simulink model "RANNSMC"  (R2017a)
settings: Solver=VariableStepAuto  StartTime=0.0  StopTime=10.0  RelTol=1e-3
undefined symbols (not defined in the file or in its folder): a21, a22
libraries: simulink x1
settings Model: Creator=ASUS  LastModifiedBy=ASUS

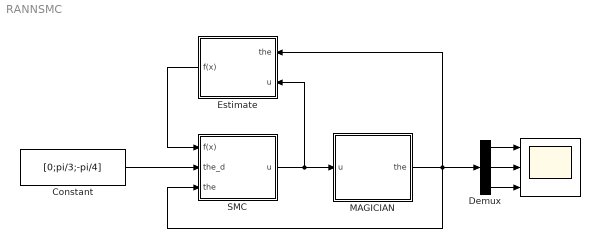
== system RANNSMC ==
  " " : Scope  NumInputPorts=3
  Constant : Constant  Value=[0;pi/3;-pi/4]
  Demux : Demux  Outputs=3
  Estimate : Subsystem
  MAGICIAN : Subsystem
  "SMC " : Subsystem
  wires:
  "SMC "/1("u ") -> MAGICIAN/1("u "), Estimate/2("u ")
  MAGICIAN/1(the) -> "SMC "/3("the "), Demux/1, Estimate/1(the)
  Demux/1 -> " "/1
  Demux/2 -> " "/2
  Demux/3 -> " "/3
  Estimate/1(f(x)) -> "SMC "/1(f(x))
  Constant/1 -> "SMC "/2(the_d)

== system RANNSMC/Estimate ==
  the : Inport
  "u " : Inport  Port=2
  Demux : Demux  Outputs=3
  Demux1 : Demux  Outputs=3
  Mux : Mux  Inputs=3
  "xx1 " : Subsystem
  "xx2 " : Subsystem
  xx3 : Subsystem
  f(x) : Outport
  wires:
  "u "/1 -> Demux1/1
  the/1 -> Demux/1
  Demux/1 -> "xx1 "/1(the1)
  Demux/2 -> "xx2 "/1(the2)
  Demux/3 -> xx3/1(the3)
  Demux1/1 -> "xx1 "/2(u1)
  Demux1/2 -> "xx2 "/2(u2)
  Demux1/3 -> xx3/2(u3)
  "xx1 "/1(f(x)1^) -> Mux/1
  xx3/1(f(x)3^) -> Mux/3
  Mux/1 -> f(x)/1
  "xx2 "/1(f(x)2^) -> Mux/2

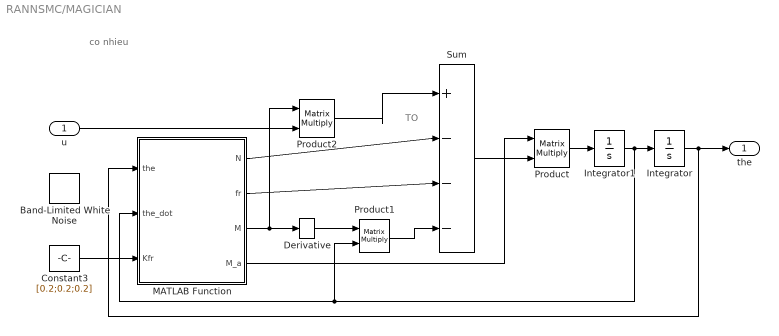
== system RANNSMC/MAGICIAN ==
  note: co nhieu
  note: TO
  "u " : Inport
  Band-Limited White Noise : simulink/Sources/Band-Limited White Noise  Cov=[0.1]  Ts=0.1  seed=[23341]
  Constant3 : Constant  Value=[0.2;0.2;0.2]
  Derivative : Derivative
  Integrator : Integrator  InitialCondition=[0;0;0]
  Integrator1 : Integrator  InitialCondition=[0;0;0]
  MATLAB Function : MATLAB Function  TreatAsAtomicUnit=on
  Product : Product  Multiplication=Matrix(*)
  Product1 : Product  Multiplication=Matrix(*)
  Product2 : Product  Multiplication=Matrix(*)
  Sum : Sum  Inputs=|+---
  the : Outport
  wires:
  Derivative/1 -> Product1/1
  Integrator1/1 -> MATLAB Function/2(the_dot), Product1/2, Integrator/1
  Product1/1 -> Sum/4
  Constant3/1 -> MATLAB Function/3(Kfr)
  MATLAB Function/3(M) -> Product2/1, Derivative/1
  Product/1 -> Integrator1/1
  MATLAB Function/2(fr) -> Sum/3
  MATLAB Function/1(N) -> Sum/2
  MATLAB Function/4(M_a) -> Product/1
  Integrator/1 -> MATLAB Function/1(the), the/1
  Sum/1 -> Product/2
  "u "/1 -> Product2/2
  Product2/1 -> Sum/1

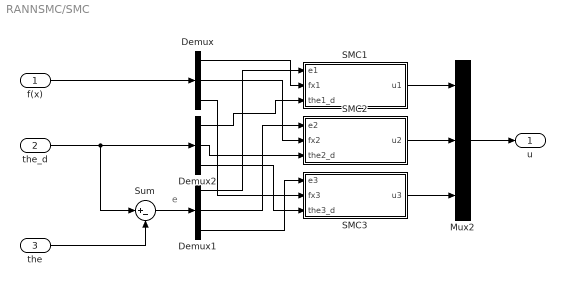
== system RANNSMC/SMC  ==
  note: e
  f(x) : Inport
  the_d : Inport  Port=2
  "the " : Inport  Port=3
  Demux : Demux  Outputs=3
  Demux1 : Demux  Outputs=3
  Demux2 : Demux  Outputs=3
  Mux2 : Mux  Inputs=3
  "SMC1 " : Subsystem
  "SMC2 " : Subsystem
  "SMC3 " : Subsystem
  Sum : Sum  Inputs=|+-
  "u " : Outport
  wires:
  "SMC1 "/1(u1) -> Mux2/1
  Mux2/1 -> "u "/1
  f(x)/1 -> Demux/1
  Demux/1 -> "SMC1 "/2(fx1)
  Demux1/1 -> "SMC1 "/1(e1)
  "SMC2 "/1(u2) -> Mux2/2
  Demux/2 -> "SMC2 "/2(fx2)
  Demux1/2 -> "SMC2 "/1(e2)
  the_d/1 -> Sum/1, Demux2/1
  Demux2/1 -> "SMC1 "/3(the1_d)
  "SMC3 "/1(u3) -> Mux2/3
  Demux1/3 -> "SMC3 "/1(e3)
  Demux/3 -> "SMC3 "/2(fx3)
  Demux2/2 -> "SMC2 "/3(the2_d)
  Demux2/3 -> "SMC3 "/3(the3_d)
  Sum/1 -> Demux1/1
  "the "/1 -> Sum/2

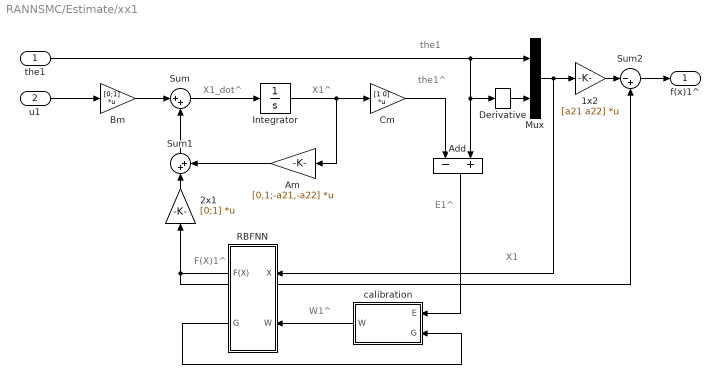
== system RANNSMC/Estimate/xx1  ==
  note: W1^
  note: the1
  note: the1^
  note: E1^
  note: X1_dot^
  note: X1^
  note: X1
  note: F(X)1^
  the1 : Inport
  u1 : Inport  Port=2
  " calibration" : Subsystem
  " RBFNN" : Subsystem
  1x2 : Gain  Gain=[a21 a22]  Multiplication=Matrix(K*u)
  2x1 : Gain  Gain=[0;1]  Multiplication=Matrix(K*u)
  Add : Sum  Inputs=-+
  "Am " : Gain  Gain=[0,1;-a21,-a22]  Multiplication=Matrix(K*u)
  Bm : Gain  Gain=[0;1]  Multiplication=Matrix(K*u)
  Cm : Gain  Gain=[1 0]  Multiplication=Matrix(K*u)
  Derivative : Derivative
  Integrator : Integrator
  Mux : Mux  Inputs=2
  Sum : Sum  Inputs=|++
  Sum1 : Sum  Inputs=|++
  Sum2 : Sum  Inputs=|-+
  f(x)1^ : Outport
  wires:
  Mux/1 -> 1x2/1, " RBFNN"/1("X ")
  Sum1/1 -> Sum/2
  u1/1 -> Bm/1
  2x1/1 -> Sum1/1
  Derivative/1 -> Mux/2
  Add/1 -> " calibration"/1(E)
  Sum/1 -> Integrator/1
  the1/1 -> Mux/1, Derivative/1, Add/2
  " calibration"/1(W) -> " RBFNN"/2(W)
  Integrator/1 -> Cm/1, "Am "/1
  "Am "/1 -> Sum1/2
  Sum2/1 -> f(x)1^/1
  " RBFNN"/2(G) -> " calibration"/2(G)
  Cm/1 -> Add/1
  1x2/1 -> Sum2/1
  Bm/1 -> Sum/1
  " RBFNN"/1(F(X)) -> 2x1/1, Sum2/2

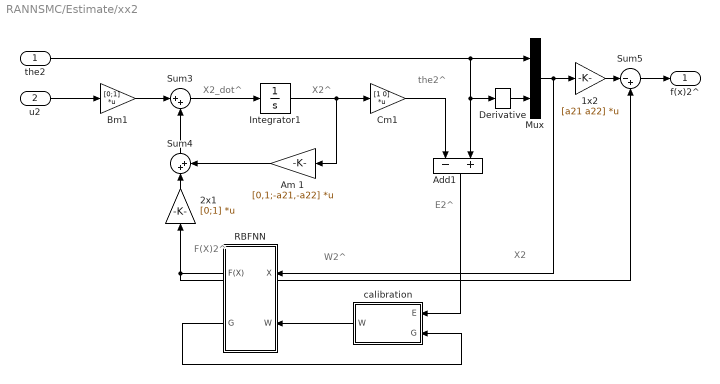
== system RANNSMC/Estimate/xx2  ==
  note: W2^
  note: the2^
  note: E2^
  note: X2_dot^
  note: X2^
  note: X2
  note: F(X)2^
  the2 : Inport
  u2 : Inport  Port=2
  " calibration" : Subsystem
  " RBFNN" : Subsystem
  1x2 : Gain  Gain=[a21 a22]  Multiplication=Matrix(K*u)
  2x1 : Gain  Gain=[0;1]  Multiplication=Matrix(K*u)
  Add1 : Sum  Inputs=-+
  Am 1 : Gain  Gain=[0,1;-a21,-a22]  Multiplication=Matrix(K*u)
  Bm1 : Gain  Gain=[0;1]  Multiplication=Matrix(K*u)
  Cm1 : Gain  Gain=[1 0]  Multiplication=Matrix(K*u)
  Derivative : Derivative
  Integrator1 : Integrator
  Mux : Mux  Inputs=2
  Sum3 : Sum  Inputs=|++
  Sum4 : Sum  Inputs=|++
  Sum5 : Sum  Inputs=|-+
  f(x)2^ : Outport
  wires:
  Mux/1 -> 1x2/1, " RBFNN"/1("X ")
  Sum4/1 -> Sum3/2
  u2/1 -> Bm1/1
  2x1/1 -> Sum4/1
  Derivative/1 -> Mux/2
  Add1/1 -> " calibration"/1(E)
  Sum3/1 -> Integrator1/1
  the2/1 -> Mux/1, Derivative/1, Add1/2
  " calibration"/1(W) -> " RBFNN"/2(W)
  Integrator1/1 -> Cm1/1, Am 1/1
  Am 1/1 -> Sum4/2
  Sum5/1 -> f(x)2^/1
  " RBFNN"/2(G) -> " calibration"/2(G)
  Cm1/1 -> Add1/1
  1x2/1 -> Sum5/1
  Bm1/1 -> Sum3/1
  " RBFNN"/1(F(X)) -> 2x1/1, Sum5/2

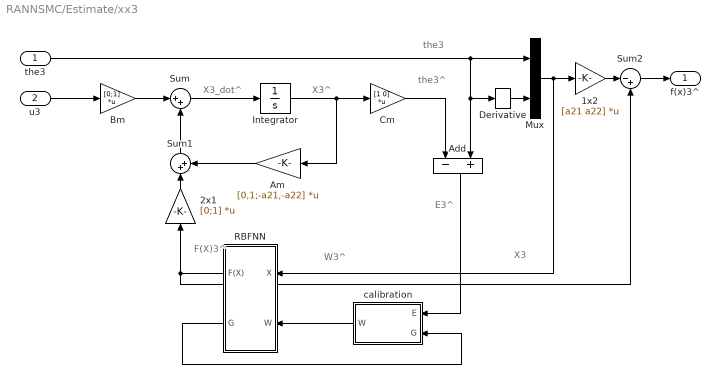
== system RANNSMC/Estimate/xx3 ==
  note: W3^
  note: X3
  note: the3
  note: the3^
  note: X3^
  note: X3_dot^
  note: F(X)3^
  note: E3^
  the3 : Inport
  u3 : Inport  Port=2
  " calibration" : Subsystem
  " RBFNN" : Subsystem
  1x2 : Gain  Gain=[a21 a22]  Multiplication=Matrix(K*u)
  2x1 : Gain  Gain=[0;1]  Multiplication=Matrix(K*u)
  Add : Sum  Inputs=-+
  "Am " : Gain  Gain=[0,1;-a21,-a22]  Multiplication=Matrix(K*u)
  Bm : Gain  Gain=[0;1]  Multiplication=Matrix(K*u)
  Cm : Gain  Gain=[1 0]  Multiplication=Matrix(K*u)
  Derivative : Derivative
  Integrator : Integrator
  Mux : Mux  Inputs=2
  Sum : Sum  Inputs=|++
  Sum1 : Sum  Inputs=|++
  Sum2 : Sum  Inputs=|-+
  f(x)3^ : Outport
  wires:
  "Am "/1 -> Sum1/2
  u3/1 -> Bm/1
  Sum/1 -> Integrator/1
  Sum2/1 -> f(x)3^/1
  " RBFNN"/1(F(X)) -> 2x1/1, Sum2/2
  Integrator/1 -> Cm/1, "Am "/1
  Add/1 -> " calibration"/1(E)
  the3/1 -> Mux/1, Derivative/1, Add/2
  Bm/1 -> Sum/1
  1x2/1 -> Sum2/1
  Sum1/1 -> Sum/2
  2x1/1 -> Sum1/1
  Derivative/1 -> Mux/2
  Cm/1 -> Add/1
  " calibration"/1(W) -> " RBFNN"/2(W)
  Mux/1 -> 1x2/1, " RBFNN"/1("X ")
  " RBFNN"/2(G) -> " calibration"/2(G)

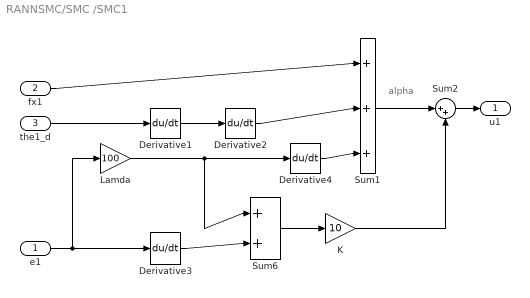
== system RANNSMC/SMC /SMC1  ==
  note: alpha
  e1 : Inport
  fx1 : Inport  Port=2
  the1_d : Inport  Port=3
  Derivative{1..4} (4 alike) : Derivative
  "K " : Gain  Gain=10
  Lamda : Gain  Gain=100
  Sum1 : Sum  Inputs=|+++
  Sum2 : Sum  Inputs=|++
  Sum6 : Sum  Inputs=|++
  u1 : Outport
  wires:
  Derivative1/1 -> Derivative2/1
  Derivative3/1 -> Sum6/2
  Sum6/1 -> "K "/1
  Sum2/1 -> u1/1
  Sum1/1 -> Sum2/1
  "K "/1 -> Sum2/2
  Lamda/1 -> Sum6/1, Derivative4/1
  Derivative4/1 -> Sum1/3
  e1/1 -> Lamda/1, Derivative3/1
  the1_d/1 -> Derivative1/1
  fx1/1 -> Sum1/1
  Derivative2/1 -> Sum1/2

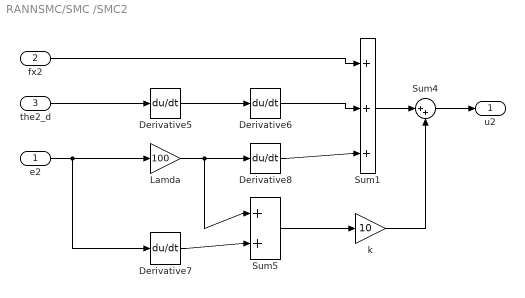
== system RANNSMC/SMC /SMC2  ==
  e2 : Inport
  fx2 : Inport  Port=2
  the2_d : Inport  Port=3
  Derivative{5..8} (4 alike) : Derivative
  Lamda : Gain  Gain=100
  Sum1 : Sum  Inputs=|+++
  Sum4 : Sum  Inputs=|++
  Sum5 : Sum  Inputs=|++
  k : Gain  Gain=10
  u2 : Outport
  wires:
  fx2/1 -> Sum1/1
  Derivative8/1 -> Sum1/3
  the2_d/1 -> Derivative5/1
  e2/1 -> Derivative7/1, Lamda/1
  Sum4/1 -> u2/1
  Lamda/1 -> Sum5/1, Derivative8/1
  Derivative5/1 -> Derivative6/1
  Sum1/1 -> Sum4/1
  Derivative7/1 -> Sum5/2
  k/1 -> Sum4/2
  Sum5/1 -> k/1
  Derivative6/1 -> Sum1/2

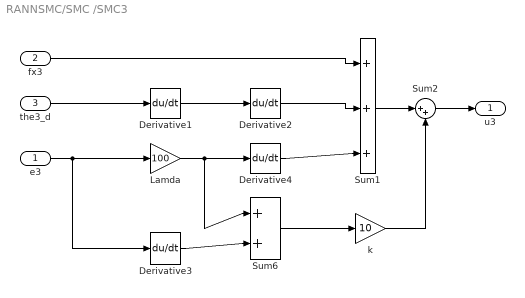
== system RANNSMC/SMC /SMC3  ==
  e3 : Inport
  fx3 : Inport  Port=2
  the3_d : Inport  Port=3
  Derivative{1..4} (4 alike) : Derivative
  Lamda : Gain  Gain=100
  Sum1 : Sum  Inputs=|+++
  Sum2 : Sum  Inputs=|++
  Sum6 : Sum  Inputs=|++
  "k " : Gain  Gain=10
  u3 : Outport
  wires:
  fx3/1 -> Sum1/1
  Derivative4/1 -> Sum1/3
  the3_d/1 -> Derivative1/1
  e3/1 -> Derivative3/1, Lamda/1
  Sum2/1 -> u3/1
  Lamda/1 -> Sum6/1, Derivative4/1
  Derivative1/1 -> Derivative2/1
  Sum1/1 -> Sum2/1
  Derivative3/1 -> Sum6/2
  "k "/1 -> Sum2/2
  Sum6/1 -> "k "/1
  Derivative2/1 -> Sum1/2

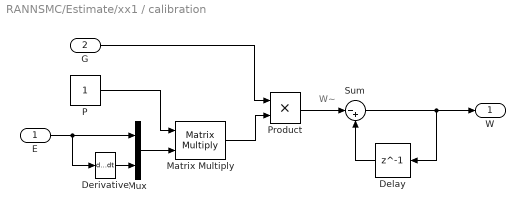
== system RANNSMC/Estimate/xx1 / calibration ==
  note: W~
  E : Inport
  G : Inport  Port=2
  Delay : Delay  DelayLength=1  InitialCondition=0
  Derivative : Derivative
  Matrix Multiply : Product  Multiplication=Matrix(*)
  Mux : Mux  Inputs=2
  P : Constant
  Product : Product
  Sum : Sum  Inputs=|-+
  W : Outport
  wires:
  E/1 -> Derivative/1, Mux/1
  Derivative/1 -> Mux/2
  Sum/1 -> W/1, Delay/1
  Delay/1 -> Sum/2
  P/1 -> Matrix Multiply/1
  Mux/1 -> Matrix Multiply/2
  Matrix Multiply/1 -> Product/2
  Product/1 -> Sum/1
  G/1 -> Product/1

== system RANNSMC/Estimate/xx1 / RBFNN ==
  "X " : Inport
  W : Inport  Port=2
  Center : Constant  Value=[1;1]
  Demux : Demux  Outputs=2
  W*Gaussian : MATLAB Function  TreatAsAtomicUnit=on
  num of neural : Constant  Value=3
  radius : Constant  Value=[0.2;0.2]
  F(X) : Outport
  G : Outport  Port=2
  wires:
  Center/1 -> W*Gaussian/3(C)
  radius/1 -> W*Gaussian/4(r)
  W*Gaussian/1(FX) -> F(X)/1
  W/1 -> W*Gaussian/5(w)
  "X "/1 -> Demux/1
  Demux/1 -> W*Gaussian/1(the)
  Demux/2 -> W*Gaussian/2(the_dot)
  num of neural/1 -> W*Gaussian/6(m)
  W*Gaussian/2(Gaussian) -> G/1

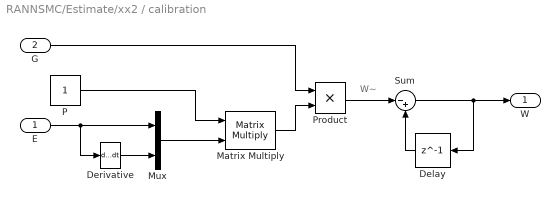
== system RANNSMC/Estimate/xx2 / calibration ==
  note: W~
  E : Inport
  G : Inport  Port=2
  Delay : Delay  DelayLength=1  InitialCondition=0
  Derivative : Derivative
  Matrix Multiply : Product  Multiplication=Matrix(*)
  Mux : Mux  Inputs=2
  P : Constant
  Product : Product
  Sum : Sum  Inputs=|-+
  W : Outport
  wires:
  E/1 -> Derivative/1, Mux/1
  Derivative/1 -> Mux/2
  Sum/1 -> Delay/1, W/1
  Delay/1 -> Sum/2
  P/1 -> Matrix Multiply/1
  Mux/1 -> Matrix Multiply/2
  Matrix Multiply/1 -> Product/2
  Product/1 -> Sum/1
  G/1 -> Product/1

== system RANNSMC/Estimate/xx2 / RBFNN ==
  "X " : Inport
  W : Inport  Port=2
  Center : Constant  Value=[1;1]
  Demux : Demux  Outputs=2
  W*Gaussian : MATLAB Function  TreatAsAtomicUnit=on
  num of neural : Constant  Value=3
  radius : Constant  Value=[0.2;0.2]
  F(X) : Outport
  G : Outport  Port=2
  wires:
  Center/1 -> W*Gaussian/3(C)
  radius/1 -> W*Gaussian/4(r)
  W*Gaussian/1(FX) -> F(X)/1
  W/1 -> W*Gaussian/5(w)
  "X "/1 -> Demux/1
  Demux/1 -> W*Gaussian/1(the)
  Demux/2 -> W*Gaussian/2(the_dot)
  num of neural/1 -> W*Gaussian/6(m)
  W*Gaussian/2(Gaussian) -> G/1

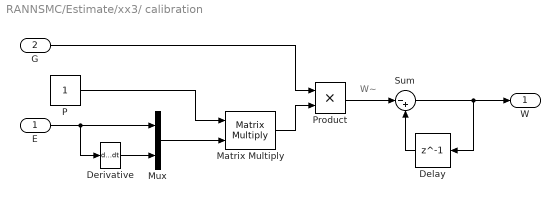
== system RANNSMC/Estimate/xx3/ calibration ==
  note: W~
  E : Inport
  G : Inport  Port=2
  Delay : Delay  DelayLength=1  InitialCondition=0
  Derivative : Derivative
  Matrix Multiply : Product  Multiplication=Matrix(*)
  Mux : Mux  Inputs=2
  P : Constant
  Product : Product
  Sum : Sum  Inputs=|-+
  W : Outport
  wires:
  E/1 -> Derivative/1, Mux/1
  Derivative/1 -> Mux/2
  Sum/1 -> Delay/1, W/1
  Delay/1 -> Sum/2
  P/1 -> Matrix Multiply/1
  Mux/1 -> Matrix Multiply/2
  Matrix Multiply/1 -> Product/2
  Product/1 -> Sum/1
  G/1 -> Product/1

== system RANNSMC/Estimate/xx3/ RBFNN ==
  "X " : Inport
  W : Inport  Port=2
  Center : Constant  Value=[1;1]
  Demux : Demux  Outputs=2
  W*Gaussian : MATLAB Function  TreatAsAtomicUnit=on
  num of neural : Constant  Value=3
  radius : Constant  Value=[0.2;0.2]
  F(X) : Outport
  G : Outport  Port=2
  wires:
  Center/1 -> W*Gaussian/3(C)
  radius/1 -> W*Gaussian/4(r)
  W*Gaussian/1(FX) -> F(X)/1
  W/1 -> W*Gaussian/5(w)
  "X "/1 -> Demux/1
  Demux/1 -> W*Gaussian/1(the)
  Demux/2 -> W*Gaussian/2(the_dot)
  num of neural/1 -> W*Gaussian/6(m)
  W*Gaussian/2(Gaussian) -> G/1

== matlab function RANNSMC/Estimate/xx1 / RBFNN/W*Gaussian ==
  data: the input; FX output; the_dot input; C input; r input; w input; m input; Gaussian output
function [FX,Gaussian]  = fcn(the,the_dot,C,r,w,m)
gauss = [0;0;0];
for i =1:m   
    mau = 0;
    for j=1:m
        bk = [the(j);the_dot(j)] - C;
        mau = mau + exp(-(bk(1)^2 + bk(2)^2)/(r(1)^2 + r(2)^2));
    end
    bk = [the(i);the_dot(i)] - C;
    gauss(i) = exp(-(bk(1)^2 + bk(2)^2)/(r(1)^2 + r(2)^2))/ mau;
end
Gaussian = [gauss(1); gauss(2); gauss(3)];
W = transpose(w);
FX = W*Gaussian;

== matlab function RANNSMC/MAGICIAN/MATLAB Function ==
  data: the input; N output; fr output; M output; M_a output; the_dot input; Kfr input
function [N,fr,M,M_a] = fcn(the,the_dot,Kfr)
the1=the(1); the2=the(2); the3=the(3);
L1 = 0.2; L2 = 0.5 ; L3= 0.5; 
m1 = 2 ; m2 = 0.3 ; m3 =0.1 ;

%DAO HAM P_0_m1 THEO THE1
J_0_m1_dot_the1 = [ 0; 0; 0];
%DAO HAM P_0_m1 THEO THE2
J_0_m1_dot_the2 = [ 0; 0; 0];
%DAO HAM P_0_m1 THEO THE3
J_0_m1_dot_the3 = [ 0; 0; 0]; 

J_0_m1 = [J_0_m1_dot_the1 J_0_m1_dot_the2 J_0_m1_dot_the3];

%DAO HAM P_0_m2 THEO THE1
J_0_m2_dot_the1 = [L2*sin(-the1)*cos(the2);L2*cos(the2)*cos(the1); 0];
%DAO HAM P_0_m2 THEO THE2
J_0_m2_dot_the2 = [L2*cos(the1)*sin(-the2);L2*sin(-the2)*sin(the1); L2*cos(the2)];
%DAO HAM P_0_m2 THEO THE3
J_0_m2_dot_the3 = [ 0; 0; 0]; 

J_0_m2 = [J_0_m2_dot_the1  J_0_m2_dot_the2  J_0_m2_dot_the3];

%DAO HAM P_0_m3 THEO THE1
J_0_m3_dot_the1 = [sin(-the1)*(L3*cos(the2 + the3) + L2*cos(the2));	 cos(the1)*(L3*cos(the2 + the3) + L2*cos(the2));     0];
%DAO HAM P_0_m3 THEO THE2
J_0_m3_dot_the2 = [cos(the1)*(L3*sin(-the2 - the3) + L2*sin(-the2));  sin(the1)*(L3*sin(-the2 - the3) + L2*sin(-the2));    L3*cos(the2 + the3) + L2*cos(the2)];
%DAO HAM P_0_m3 THEO THE3
J_0_m3_dot_the3 = [ cos(the1)*L3*sin(-the2 - the3);	 sin(the1)*L3*sin(-the2 - the3);  L3*cos(the2 + the3)];

J_0_m3 = [J_0_m3_dot_the1  J_0_m3_dot_the2  J_0_m3_dot_the3];

% % % % % % % % % % % % % % % % % % % % % % % % 
%TONG HOP MA TRAN M3
M3 = (m3*[0 0 1]*transpose(J_0_m3)*J_0_m3);

%TONG HOP MA TRAN M2
M2 = (m2*[0 1 0]*transpose(J_0_m2)*J_0_m2 + m3*[0 1 0]*transpose(J_0_m3)*J_0_m3); 

%TONG HOP MA TRAN M1
M1 = (m1*[1 0 0]*transpose(J_0_m1)*J_0_m1 + m2*[1 0 0]*transpose(J_0_m2)*J_0_m2 + m3*[1 0 0]*transpose(J_0_m2)*J_0_m3);
M  = [ M1 ; M2 ; M3];
M_a = inv(M);

%%%%%%%%%%%%%%%%%%%%%%%%%%%%%%%%%%%%%%%%%%%%%%%%%%%%%% 
%DAO HAM J_0_m1_dot_the1 theo the1
J_0_m1_dot_the1_dot_the1 = [ 0; 0; 0];
%DAO HAM J_0_m1_dot_the2 theo the1
J_0_m1_dot_the2_dot_the1 = [ 0; 0; 0];  
%DAO HAM J_0_m1_dot_the3 theo the1
J_0_m1_dot_the3_dot_the1 = [ 0; 0; 0]; 

%DAO HAM J_0_m1 theo the1 
J_0_m1_dot_the1_1 = [J_0_m1_dot_the1_dot_the1  J_0_m1_dot_the2_dot_the1  J_0_m1_dot_the3_dot_the1];

%%%%%%%%%%%%%%%%%%%%%%%%%%%%%%%%%%%%%%%%%%%%%%%%%%%%%%%%%%
%DAO HAM J_0_m2_dot_the1 theo the1
%J_0_m2_dot_the1 = [L2*sin(-the1)*cos(the2);    L2*cos(the2)*cos(the1);  0];
J_0_m2_dot_the1_dot_the1 = [L2*cos(the1)*cos(the2);L2*cos(the2)*sin(-the1); 0];
%DAO HAM J_0_m2_dot_the2 theo the1
%J_0_m2_dot_the2 = [L2*cos(the1)*sin(-the2);    L2*sin(-the2)*sin(the1);     L2*cos(the2)];
J_0_m2_dot_the2_dot_the1 = [L2*sin(the1)*sin(the2);L2*sin(-the2)*cos(the1); 0];
%DAO HAM J_0_m2_dot_the3 theo the1
J_0_m2_dot_the3_dot_the1 = [ 0; 0; 0]; 

%DAO HAM J_0_m2 theo the1 
J_0_m2_dot_the1_1 = [J_0_m2_dot_the1_dot_the1   J_0_m2_dot_the2_dot_the1  J_0_m2_dot_the3_dot_the1];

%%%%%%%%%%%%%%%%%%%%%%%%%%%%%%%%%%%%%%%%%%%%%%%%%%%%%%%%%%%
%DAO HAM J_0_m2_dot_the1 theo the2
%J_0_m2_dot_the1 = [L2*sin(-the1)*cos(the2);    L2*cos(the2)*cos(the1);  0];
J_0_m2_dot_the1_dot_the2 = [L2*sin(the1)*sin(the2);L2*sin(-the2)*cos(the1); 0];
%DAO HAM J_0_m2_dot_the2 theo the2
%J_0_m2_dot_the2 = [L2*cos(the1)*sin(-the2);    L2*sin(-the2)*sin(the1);     L2*cos(the2)];
J_0_m2_dot_the2_dot_the2 = [L2*cos(the1)*cos(the2);L2*cos(the2)*sin(the1); L2*sin(-the2)];
%DAO HAM J_0_m2_dot_the3 theo the2
J_0_m2_dot_the3_dot_the2 = [ 0; 0; 0]; 

%DAO HAM J_0_m2 theo the2
J_0_m2_dot_the2_2 = [J_0_m2_dot_the1_dot_the2  J_0_m2_dot_the2_dot_the2  J_0_m2_dot_the3_dot_the2];

%%%%%%%%%%%%%%%%%%%%%%%%%%%%%%%%%%%%%%%%%%%%%%%%%%%%%%%%%%%%%%%
%DAO HAM J_0_m3_dot_the1 theo the1
%J_0_m3_dot_the1 = [sin(-the1)*(L3*cos(the2 + the3) + L2*cos(the2));	 cos(the1)*(L3*cos(the2 + the3) + L2*cos(the2));     0];
J_0_m3_dot_the1_dot_the1 = [cos(the1)*(L3*cos(the2 + the3) + L2*cos(the2));	 sin(-the1)*(L3*cos(the2 + the3) + L2*cos(the2));     0];
%DAO HAM J_0_m3_dot_the2 theo the1
%J_0_m3_dot_the2 =          [cos(the1)*(L3*sin(-the2 - the3) + L2*sin(-the2));  sin(the1)*(L3*sin(-the2 - the3) + L2*sin(-the2));    L3*cos(the2 + the3) + L2*cos(the2)];
J_0_m3_dot_the2_dot_the1 = [sin(the1)*(L3*sin(the2 + the3) + L2*sin(the2));  -cos(the1)*(L3*sin(the2 + the3) + L2*sin(the2));    0];
%DAO HAM J_0_m3_dot_the3 theo the1
%J_0_m3_dot_the3 =          [ cos(the1)*L3*sin(-the2 - the3);	 sin(the1)*L3*sin(-the2 - the3);  L3*cos(the2 + the3)];
J_0_m3_dot_the3_dot_the1 = [ sin(the1)*L3*sin(the2 + the3);     -cos(the1)*L3*sin(the2 + the3);  0];

J_0_m3_dot_the1_1 = [J_0_m3_dot_the1_dot_the1  J_0_m3_dot_the2_dot_the1  J_0_m3_dot_the3_dot_the1];

%%%%%%%%%%%%%%%%%%%%%%%%%%%%%%%%%%%%%%%%%%%%%%%%%%%%%%%%%%%%%

%DAO HAM J_0_m3_dot_the1 theo the2
%J_0_m3_dot_the1 =          [sin(-the1)*(L3*cos(the2 + the3) + L2*cos(the2));	 cos(the1)*(L3*cos(the2 + the3) + L2*cos(the2));     0];
J_0_m3_dot_the1_dot_the2 = [sin(the1)*(L3*sin(the2 + the3) + L2*sin(the2));	 -cos(the1)*(L3*sin(the2 + the3) + L2*sin(the2));     0];
%DAO HAM J_0_m3_dot_the2 theo the2
%J_0_m3_dot_the2 =        [cos(the1)*(L3*sin(-the2 - the3) + L2*sin(-the2));  sin(the1)*(L3*sin(-the2 - the3) + L2*sin(-the2));    L3*cos(the2 + the3) + L2*cos(the2)];
J_0_m3_dot_the2_dot_the2 = [cos(the1)*(L3*cos(the2 + the3) + L2*cos(the2));  sin(the1)*(L3*cos(the2 + the3) + L2*cos(the2));    -L3*sin(the2 + the3) - L2*sin(the2)];
%DAO HAM J_0_m3_dot_the3 theo the2
%J_0_m3_dot_the3 =         [ cos(the1)*L3*sin(-the2 - the3);	 sin(the1)*L3*sin(-the2 - the3);  L3*cos(the2 + the3)];
J_0_m3_dot_the3_dot_the2 = [ cos(the1)*L3*cos(the2 + the3);     sin(the1)*L3*cos(the2 + the3);  -L3*sin(the2 + the3)];

%DAO HAM J_0_m3 theo the2
J_0_m3_dot_the2_2= [J_0_m3_dot_the1_dot_the2  J_0_m3_dot_the2_dot_the2  J_0_m3_dot_the3_dot_the2];
 

%%%%%%%%%%%%%%%%%%%%%%%%%%%%%%%%%%%%%%%%%%%%%%%%%%%%%%%%%%%%%
%DAO HAM J_0_m3_dot_the1 theo the3
%J_0_m3_dot_the1 =         [sin(-the1)*(L3*cos(the2 + the3) + L2*cos(the2));	 cos(the1)*(L3*cos(the2 + the3) + L2*cos(the2));     0];
J_0_m3_dot_the1_dot_the3 = [sin(the1)*L3*sin(the2 + the3);	 -cos(the1)*L3*sin(the2 + the3);     0];
%DAO HAM J_0_m3_dot_the2 theo the3
%J_0_m3_dot_the2 =        [cos(the1)*(L3*sin(-the2 - the3) + L2*sin(-the2));  sin(the1)*(L3*sin(-the2 - the3) + L2*sin(-the2));    L3*cos(the2 + the3) + L2*cos(the2)];
J_0_m3_dot_the2_dot_the3 = [cos(the1)*L3*cos(the2 + the3);  sin(the1)*L3*cos(the2 + the3);    -L3*sin(the2 + the3)];
%DAO HAM J_0_m3_dot_the3 theo the3
%J_0_m3_dot_the3 =         [ cos(the1)*L3*sin(-the2 - the3);	 sin(the1)*L3*sin(-the2 - the3);  L3*cos(the2 + the3)];
J_0_m3_dot_the3_dot_the3 = [ cos(the1)*L3*cos(the2 + the3);	 sin(the1)*L3*cos(the2 + the3);  -L3*sin(the2 + the3)];

%DAO HAM J_0_m3 theo the3
J_0_m3_dot_the3_3 = [J_0_m3_dot_the1_dot_the3 J_0_m3_dot_the2_dot_the3  J_0_m3_dot_the3_dot_the3];
 
%%%%%%%%%%%%%%%%%%%%%%%%%%%%%%%%%%%%%%%%%%
dT_dthe3 = transpose(the_dot)*(m3*transpose(J_0_m3_dot_the3_3)*J_0_m3)*the_dot;
%%%%%%%%%%%%%%%%%%%%%%%%%%%%%%%%%%%%%%%%%%%%
dT_dthe2 = transpose(the_dot)*(m2*transpose(J_0_m2_dot_the2_2)*J_0_m2+m3*transpose(J_0_m3_dot_the2_2)*J_0_m3)*the_dot;
%%%%%%%%%%%%%%%%%%%%%%%%%%%%%%%%%%%%%%%%%%
dT_dthe1 = (transpose(the_dot)*(m1*transpose(J_0_m1_dot_the1_1)*J_0_m1+m2*transpose(J_0_m2_dot_the1_1)*J_0_m2+m3*transpose(J_0_m3_dot_the1_1)*J_0_m3)*the_dot);

%TINH dU_DTHE3
%%%%%%%%%%%%%%%%%%%%%%%%%%%%%%%%%%%%%%%%%%%%%%%%%%%%%%%%%%%%%%%
g_0 = [ 0;0;-9.81];

dU_dthe3 = -m3*transpose(g_0)*J_0_m3_dot_the3 ;
 
N3 = -dT_dthe3 + dU_dthe3;
%V3 = simplify(-dT_dthe3+M3_dot_t*the_dot)

%TINH dU_DTHE2
%%%%%%%%%%%%%%%%%%%%%%%%%%%%%%%%%%%%%%%%%%%%%%%%%%%%%%%%%%%%%%%
g_0 = [ 0;0;-9.81];

dU_dthe2 = -m2*transpose(g_0)*J_0_m2_dot_the2 - m3*transpose(g_0)*J_0_m3_dot_the2 ;
 
N2= -dT_dthe2 + dU_dthe2;
%V2 = simplify(-dT_dthe2 + M2_dot_t*the_dot)

%TINH dU_DTHE1
%%%%%%%%%%%%%%%%%%%%%%%%%%%%%%%%%%%%%%%%%%%%%%%%%%%%%%%%%%%%%%%
g_0 = [ 0;0;-9.81];

dU_dthe1 = -m1*transpose(g_0)*J_0_m1_dot_the1-m2*transpose(g_0)*J_0_m2_dot_the1-m3*transpose(g_0)*J_0_m3_dot_the1 ;
 
N1= -dT_dthe1  + dU_dthe1;
%V1 = simplify(-dT_dthe1+M1_dot_t*the_dot)
N = [ N1;N2;N3] ;
% I = [10;10;10];
fr = [(Kfr(1)*the_dot(1)); (Kfr(2)*the_dot(2)) ; (Kfr(3)*the_dot(3))];

== matlab function RANNSMC/Estimate/xx3/ RBFNN/W*Gaussian ==
  data: the input; FX output; the_dot input; C input; r input; w input; m input; Gaussian output
function [FX,Gaussian]  = fcn(the,the_dot,C,r,w,m)
gauss = [0;0;0];
for i =1:m   
    mau = 0;
    for j=1:m
        bk = [the(j);the_dot(j)] - C;
        mau = mau + exp(-(bk(1)^2 + bk(2)^2)/(r(1)^2 + r(2)^2));
    end
    bk = [the(i);the_dot(i)] - C;
    gauss(i) = exp(-(bk(1)^2 + bk(2)^2)/(r(1)^2 + r(2)^2))/ mau;
end
Gaussian = [gauss(1); gauss(2); gauss(3)];
W = transpose(w);
FX = W*Gaussian;

== matlab function RANNSMC/Estimate/xx2 / RBFNN/W*Gaussian ==
  data: the input; FX output; the_dot input; C input; r input; w input; m input; Gaussian output
function [FX,Gaussian]  = fcn(the,the_dot,C,r,w,m)
gauss = [0;0;0];
for i =1:m   
    mau = 0;
    for j=1:m
        bk = [the(j);the_dot(j)] - C;
        mau = mau + exp(-(bk(1)^2 + bk(2)^2)/(r(1)^2 + r(2)^2));
    end
    bk = [the(i);the_dot(i)] - C;
    gauss(i) = exp(-(bk(1)^2 + bk(2)^2)/(r(1)^2 + r(2)^2))/ mau;
end
Gaussian = [gauss(1); gauss(2); gauss(3)];
W = transpose(w);
FX = W*Gaussian;
